simulink model "sampleModel1685"  (R2023a)
settings: Solver=VariableStepAuto  StartTime=0.0  StopTime=10.0  RelTol=1e-3
libraries: hdlsllib x4, simulink x2
settings Model: Creator=user1  LastModifiedBy=user1

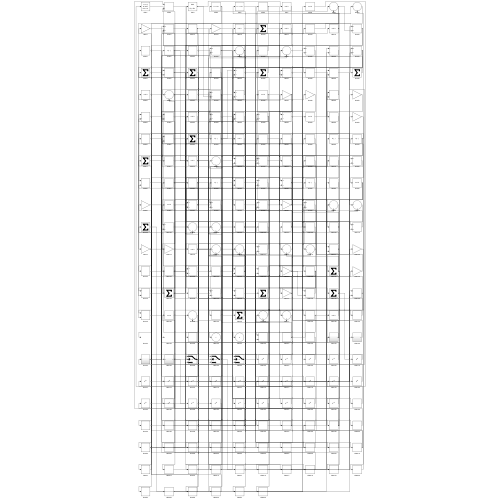
[thumbnail: Simulink's stored preview of the top-level diagram]
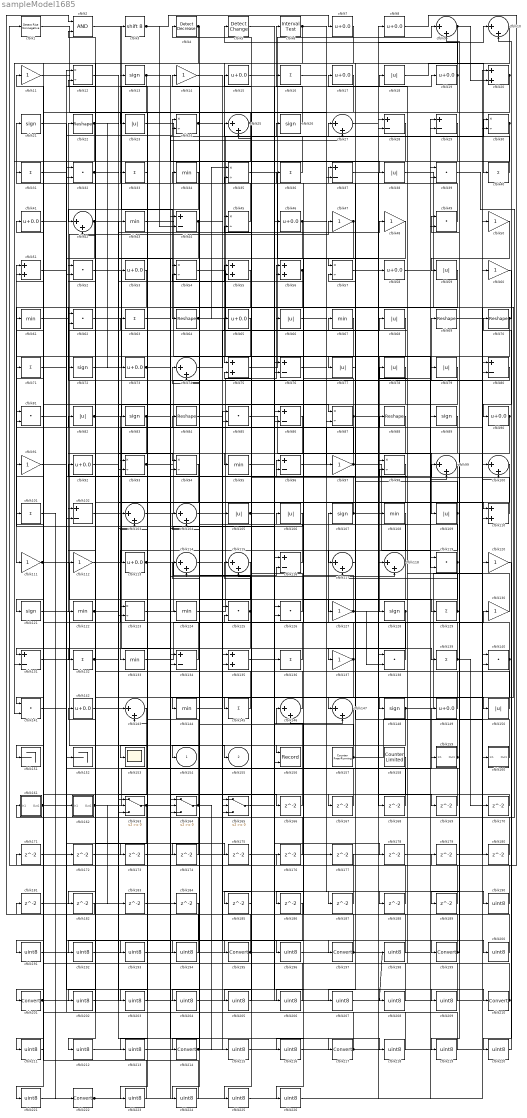
== system sampleModel1685 ==
  cfblk1 : hdlsllib/Logic and Bit Operations/Detect Rise Nonnegative  vinit=0  OutDataTypeStr=boolean
  cfblk{9..10,25,27,42,74,99..100,103..104,114..115,117..118,143,146..147} (17 alike) : Sum  Inputs=|++
  cfblk{16,31,33,36,40,63,71,101,129,132,136,139,145} (13 alike) : Sum  Inputs=+
  cfblk{28..29,37,44,76,80,86,96,102,116,131,134} (12 alike) : Sum  Inputs=+-
  cfblk{18,23,38,59,66,68,77..79,82,105..106,109,150} (14 alike) : Abs  SaturateOnIntegerOverflow=off
  cfblk{13,21,26,72,83,89,107,121,128,148} (10 alike) : Signum
  cfblk{34,43,61,67,95,108,122,124,133,144} (10 alike) : MinMax
  cfblk{11,14,47..48,50,60,91,97,111..112,120,127,130,137} (14 alike) : Gain
  cfblk{20,51,55..56,75,110,135} (7 alike) : Sum
  cfblk{7..8,15,17,19,41,46,53,58,65,73,90,92,113,142,149} (16 alike) : Bias  Bias=0.0  SaturateOnIntegerOverflow=off
  cfblk{32,39,49,52,62,81,85,119,125..126,138,140..141} (13 alike) : DotProduct  OutDataTypeStr=Inherit: Inherit via internal rule
  cfblk{12,24,30,35,45,54,57,87,93..94,98,123} (12 alike) : Product  Inputs=*/  RndMeth=Zero  SaturateOnIntegerOverflow=on
  cfblk151 : Terminator
  cfblk152 : Terminator
  cfblk153 : Scope
  cfblk156 : Record  FileSettingsInternal="{\"entries\":[{\"content\":{\"excelSettings\":{\"content\":{},\"type\":\"Streamout.ExcelSettings\"}},\"type\":\"Streamout.FileSettingStorage\",\"uuid\":\"\"}],\"packageUris\":[\"http:\\/\\/schema.mathworks.com\\/mf0\\/streamout_blocks\\/R2020a\"],\"version\":\"1.0\"}"  Layout=[1 1]  SignalsInternal="{\"entries\":[{\"content\":{\"signals\":[{\"content\":{\"blockPath\":[],\"dimensions\":[1],\"domain\":\"\",\"lineColor\":\"#a2142f\",\"plots\":[1],\"port\":1,\"signalID\":2927,\"signalName\":\"XY Graph:1\"},\"type\":\"RecordBlkView.Signal\",\"uuid\":\"\"},{\"content\":{\"blockPath\":[],\"dimensions\":[1],\"domain\":\"\",\"lineColor\":\"#139fff\",\"plots\":[1],\"port\":2,\"signalID\":2930,\"signalName\":\"XY Graph:2\"},\"type\":\"RecordBlkView.Signal\",\"uuid\":\"\"}]},\"type\":\"RecordBlkView.InputSignals\",\"uuid\":\"\"}],\"packageUris\":[\"http:\\/\\/schema.mathworks.com\\/mf0\\/streamout_blocks\\/R2020a\"],\"version\":\"1.0\"}"  VisualizationBindings="{\"xyplotplugin\":{\"info\":[{\"series\":[{\"bindingParametersList\":[{\"parameter\":\"X-Axis\",\"signalID\":2927,\"signalName\":\"XY Graph:1\"},{\"parameter\":\"Y-Axis\",\"signalID\":2930,\"signalName\":\"XY Graph:2\"}],\"seriesID\":20328}],\"subplotID\":1}]}}"  CompatibilityTag=XY  st=-1
  cfblk157 : hdlsllib/Sources/Counter Free-Running  NumBits=16  tsamp=-1
  cfblk158 : hdlsllib/Sources/Counter Limited  uplimit=7  tsamp=-1
  cfblk159 : Subsystem
      settings: LibrarySourceBlock=|
      | hdlsllib/Ports &
      | Subsystems/Subsystem
  cfblk160 : Subsystem
      settings: LibrarySourceBlock=|
      | hdlsllib/Ports &
      | Subsystems/Subsystem
  cfblk161 : Subsystem
      settings: LibrarySourceBlock=|
      | hdlsllib/Ports &
      | Subsystems/Subsystem
  cfblk162 : Subsystem
      settings: LibrarySourceBlock=|
      | hdlsllib/Ports &
      | Subsystems/Subsystem
  cfblk163 : Switch  SaturateOnIntegerOverflow=off  InputSameDT=off
  cfblk164 : Switch  SaturateOnIntegerOverflow=off  InputSameDT=off
  cfblk165 : Switch  SaturateOnIntegerOverflow=off  InputSameDT=off
  cfblk{166..189} (24 alike) : Delay  SampleTime=1
  cfblk{190..194,196,198,200,202..209,211..213,215..216,218..221,223..226} (29 alike) : DataTypeConversion  OutDataTypeStr=uint8  SaturateOnIntegerOverflow=off  RndMeth=Floor
  cfblk{195,197,199,201,210,214,217,222} (8 alike) : DataTypeConversion  SaturateOnIntegerOverflow=off  RndMeth=Floor
  cfblk2 : Logic  AllPortsSameDT=off  OutDataTypeStr=boolean
  cfblk{22,64,69..70,84,88} (6 alike) : Reshape
  cfblk3 : ArithShift  BitShiftNumber=8
  cfblk4 : simulink/Logic and Bit Operations/Detect Decrease  vinit=0.0  OutDataTypeStr=boolean
      settings: LibrarySourceBlock=|
      | hdlsllib/Logic and Bit
      | Operations/Detect
      | Decrease
  cfblk5 : simulink/Logic and Bit Operations/Detect Change  vinit=0  OutDataTypeStr=boolean
      settings: LibrarySourceBlock=|
      | hdlsllib/Logic and Bit
      | Operations/Detect
      | Change
  cfblk6 : hdlsllib/Logic and Bit Operations/Interval Test  IntervalClosedRight=on  uplimit=0.5  IntervalClosedLeft=on  lowlimit=-0.5  OutDataTypeStr=boolean
  cfblk154 : Outport  VectorParamsAs1DForOutWhenUnconnected=off
  cfblk155 : Outport  Port=2  VectorParamsAs1DForOutWhenUnconnected=off
  wires:
  cfblk72/1 -> cfblk19/1
  cfblk80/1 -> cfblk22/1
  cfblk6/1 -> cfblk75/1, cfblk110/2
  cfblk29/1 -> cfblk214/1
  cfblk18/1 -> cfblk40/1
  cfblk109/1 -> cfblk133/1, cfblk57/2
  cfblk12/1 -> cfblk217/1
  cfblk38/1 -> cfblk144/1
  cfblk159/1(Out1) -> cfblk96/1, cfblk62/2
  cfblk106/1 -> cfblk51/1
  cfblk121/1 -> cfblk155/1
  cfblk75/1 -> cfblk9/1
  cfblk103/1 -> cfblk60/1
  cfblk60/1 -> cfblk90/1
  cfblk64/1 -> cfblk30/1, cfblk35/1
  cfblk70/1 -> cfblk128/1, cfblk10/2, cfblk205/1
  cfblk82/1 -> cfblk87/1, cfblk94/1
  cfblk56/1 -> cfblk153/1, cfblk54/2
  cfblk131/1 -> cfblk47/1
  cfblk124/1 -> cfblk56/1
  cfblk85/1 -> cfblk109/1
  cfblk61/1 -> cfblk122/1
  cfblk143/1 -> cfblk201/1
  cfblk160/1(Out1) -> cfblk49/1
  cfblk52/1 -> cfblk110/1
  cfblk118/1 -> cfblk106/1, cfblk216/1
  cfblk137/1 -> cfblk107/1, cfblk182/1
  cfblk1/1 -> cfblk97/1
  cfblk17/1 -> cfblk151/1
  cfblk23/1 -> cfblk135/1
  cfblk34/1 -> cfblk132/1
  cfblk54/1 -> cfblk119/1
  cfblk46/1 -> cfblk150/1, cfblk85/2
  cfblk133/1 -> cfblk130/1
  cfblk84/1 -> cfblk165/1
  cfblk105/1 -> cfblk18/1, cfblk68/1
  cfblk71/1 -> cfblk197/1
  cfblk97/1 -> cfblk119/2, cfblk2/2
  cfblk2/1 -> cfblk64/1
  cfblk101/1 -> cfblk222/1
  cfblk25/1 -> cfblk135/2, cfblk23/1, cfblk223/1
  cfblk87/1 -> cfblk56/2, cfblk79/1, cfblk186/1
  cfblk58/1 -> cfblk39/1
  cfblk88/1 -> cfblk145/1
  cfblk49/1 -> cfblk21/1
  cfblk41/1 -> cfblk210/1
  cfblk53/1 -> cfblk111/1
  cfblk145/1 -> cfblk52/1
  cfblk99/1 -> cfblk118/1
  cfblk140/1 -> cfblk15/1, cfblk194/1
  cfblk157/1 -> cfblk140/2, cfblk84/1
  cfblk114/1 -> cfblk165/2
  cfblk93/1 -> cfblk69/1, cfblk63/1
  cfblk40/1 -> cfblk26/1
  cfblk148/1 -> cfblk50/1, cfblk165/3
  cfblk62/1 -> cfblk164/1
  cfblk134/1 -> cfblk83/1
  cfblk50/1 -> cfblk59/1
  cfblk126/1 -> cfblk4/1
  cfblk31/1 -> cfblk162/1(In1)
  cfblk142/1 -> cfblk199/1
  cfblk44/1 -> cfblk52/2, cfblk148/1, cfblk94/2
  cfblk129/1 -> cfblk62/1, cfblk117/2, cfblk189/1
  cfblk5/1 -> cfblk136/1
  cfblk128/1 -> cfblk125/2, cfblk156/2, cfblk185/1
  cfblk149/1 -> cfblk78/1
  cfblk73/1 -> cfblk147/1, cfblk118/2
  cfblk26/1 -> cfblk6/1
  cfblk136/1 -> cfblk91/1
  cfblk74/1 -> cfblk66/1
  cfblk163/1 -> cfblk27/2, cfblk202/1
  cfblk55/1 -> cfblk121/1
  cfblk43/1 -> cfblk100/1
  cfblk161/1(Out1) -> cfblk99/1, cfblk24/2
  cfblk130/1 -> cfblk17/1
  cfblk119/1 -> cfblk67/1, cfblk156/1
  cfblk67/1 -> cfblk154/1
  cfblk146/1 -> cfblk123/1
  cfblk122/1 -> cfblk48/1, cfblk129/1
  cfblk123/1 -> cfblk86/2
  cfblk125/1 -> cfblk31/1, cfblk35/2, cfblk211/1
  cfblk112/1 -> cfblk58/1
  cfblk30/1 -> cfblk45/1, cfblk57/1, cfblk131/2
  cfblk91/1 -> cfblk152/1
  cfblk45/1 -> cfblk3/1
  cfblk107/1 -> cfblk8/1, cfblk93/1
  cfblk19/1 -> cfblk95/1, cfblk5/1
  cfblk102/1 -> cfblk80/2
  cfblk83/1 -> cfblk124/1, cfblk112/1
  cfblk138/1 -> cfblk34/1
  cfblk135/1 -> cfblk147/2
  cfblk13/1 -> cfblk38/1, cfblk93/2
  cfblk141/1 -> cfblk16/1
  cfblk90/1 -> cfblk146/2, cfblk117/1, cfblk219/1
  cfblk117/1 -> cfblk37/1
  cfblk96/1 -> cfblk88/1
  cfblk89/1 -> cfblk195/1
  cfblk14/1 -> cfblk77/1
  cfblk59/1 -> cfblk72/1
  cfblk132/1 -> cfblk53/1, cfblk55/2
  cfblk24/1 -> cfblk105/1, cfblk188/1
  cfblk35/1 -> cfblk108/1
  cfblk110/1 -> cfblk65/1
  cfblk11/1 -> cfblk116/1
  cfblk39/1 -> cfblk161/1(In1)
  cfblk47/1 -> cfblk196/1, cfblk206/1
  cfblk162/1(Out1) -> cfblk149/1, cfblk183/1
  cfblk139/1 -> cfblk36/1, cfblk170/1
  cfblk9/1 -> cfblk37/2, cfblk131/1, cfblk20/2
  cfblk86/1 -> cfblk102/1
  cfblk77/1 -> cfblk127/1
  cfblk48/1 -> cfblk123/2
  cfblk20/1 -> cfblk173/1, cfblk174/1
  cfblk68/1 -> cfblk81/1
  cfblk100/1 -> cfblk164/3
  cfblk66/1 -> cfblk139/1
  cfblk113/1 -> cfblk116/2, cfblk27/1, cfblk55/1
  cfblk32/1 -> cfblk113/1, cfblk104/2
  cfblk3/1 -> cfblk7/1, cfblk44/2
  cfblk27/1 -> cfblk10/1
  cfblk22/1 -> cfblk32/2, cfblk87/2, cfblk73/1
  cfblk127/1 -> cfblk138/1, cfblk96/2, cfblk138/2
  cfblk7/1 -> cfblk42/1
  cfblk51/1 -> cfblk24/1
  cfblk4/1 -> cfblk74/2, cfblk141/2
  cfblk36/1 -> cfblk25/1
  cfblk164/1 -> cfblk81/2, cfblk215/1
  cfblk150/1 -> cfblk13/1
  cfblk116/1 -> cfblk92/1
  cfblk78/1 -> cfblk137/1
  cfblk111/1 -> cfblk134/1, cfblk141/1
  cfblk42/1 -> cfblk54/1, cfblk103/2, cfblk102/2
  cfblk92/1 -> cfblk166/1
  cfblk166/1 -> cfblk45/2
  cfblk10/1 -> cfblk167/1
  cfblk167/1 -> cfblk42/2
  cfblk37/1 -> cfblk168/1
  cfblk168/1 -> cfblk86/1
  cfblk57/1 -> cfblk169/1
  cfblk169/1 -> cfblk32/1
  cfblk170/1 -> cfblk164/2
  cfblk171/1 -> cfblk39/2
  cfblk21/1 -> cfblk172/1
  cfblk172/1 -> cfblk30/2
  cfblk173/1 -> cfblk99/2
  cfblk174/1 -> cfblk163/2
  cfblk81/1 -> cfblk175/1
  cfblk175/1 -> cfblk100/2
  cfblk176/1 -> cfblk104/1
  cfblk16/1 -> cfblk177/1
  cfblk177/1 -> cfblk1/1
  cfblk95/1 -> cfblk178/1
  cfblk178/1 -> cfblk80/1
  cfblk8/1 -> cfblk179/1
  cfblk179/1 -> cfblk9/2
  cfblk69/1 -> cfblk180/1
  cfblk180/1 -> cfblk51/2
  cfblk181/1 -> cfblk163/3
  cfblk182/1 -> cfblk2/1
  cfblk183/1 -> cfblk134/2
  cfblk185/1 -> cfblk75/2
  cfblk144/1 -> cfblk187/1
  cfblk187/1 -> cfblk146/1
  cfblk188/1 -> cfblk103/1
  cfblk189/1 -> cfblk61/1
  cfblk76/1 -> cfblk190/1
  cfblk190/1 -> cfblk126/1
  cfblk65/1 -> cfblk191/1
  cfblk191/1 -> cfblk76/1
  cfblk94/1 -> cfblk192/1
  cfblk192/1 -> cfblk76/2
  cfblk33/1 -> cfblk193/1
  cfblk193/1 -> cfblk126/2
  cfblk194/1 -> cfblk33/1
  cfblk195/1 -> cfblk163/1, cfblk85/1
  cfblk196/1 -> cfblk89/1
  cfblk197/1 -> cfblk176/1, cfblk82/1
  cfblk198/1 -> cfblk71/1
  cfblk199/1 -> cfblk159/1(In1), cfblk25/2, cfblk14/1
  cfblk104/1 -> cfblk200/1
  cfblk200/1 -> cfblk142/1
  cfblk201/1 -> cfblk198/1, cfblk46/1, cfblk43/1
  cfblk202/1 -> cfblk143/1
  cfblk186/1 -> cfblk203/1
  cfblk203/1 -> cfblk143/2
  cfblk115/1 -> cfblk204/1
  cfblk204/1 -> cfblk114/1
  cfblk205/1 -> cfblk115/1
  cfblk206/1 -> cfblk115/2
  cfblk98/1 -> cfblk207/1
  cfblk207/1 -> cfblk160/1(In1)
  cfblk165/1 -> cfblk208/1
  cfblk208/1 -> cfblk98/1
  cfblk15/1 -> cfblk209/1
  cfblk209/1 -> cfblk98/2
  cfblk210/1 -> cfblk44/1, cfblk11/1
  cfblk211/1 -> cfblk41/1
  cfblk184/1 -> cfblk212/1
  cfblk212/1 -> cfblk125/1
  cfblk108/1 -> cfblk213/1
  cfblk213/1 -> cfblk184/1
  cfblk214/1 -> cfblk20/1, cfblk74/1
  cfblk215/1 -> cfblk29/1
  cfblk216/1 -> cfblk29/2
  cfblk217/1 -> cfblk181/1, cfblk140/1
  cfblk63/1 -> cfblk218/1
  cfblk218/1 -> cfblk12/1
  cfblk219/1 -> cfblk12/2
  cfblk120/1 -> cfblk220/1
  cfblk220/1 -> cfblk70/1
  cfblk79/1 -> cfblk221/1
  cfblk221/1 -> cfblk120/1
  cfblk222/1 -> cfblk114/2, cfblk49/2
  cfblk223/1 -> cfblk101/1
  cfblk28/1 -> cfblk224/1
  cfblk224/1 -> cfblk171/1
  cfblk158/1 -> cfblk225/1
  cfblk225/1 -> cfblk28/1
  cfblk147/1 -> cfblk226/1
  cfblk226/1 -> cfblk28/2

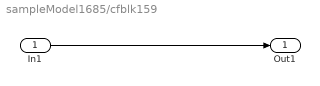
== system sampleModel1685/cfblk159 ==
  In1 : Inport
  Out1 : Outport
  wires:
  In1/1 -> Out1/1

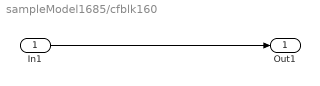
== system sampleModel1685/cfblk160 ==
  In1 : Inport
  Out1 : Outport
  wires:
  In1/1 -> Out1/1

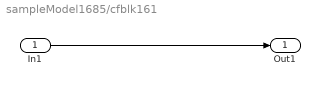
== system sampleModel1685/cfblk161 ==
  In1 : Inport
  Out1 : Outport
  wires:
  In1/1 -> Out1/1

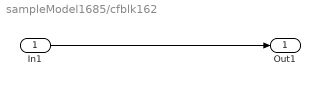
== system sampleModel1685/cfblk162 ==
  In1 : Inport
  Out1 : Outport
  wires:
  In1/1 -> Out1/1
